simulink model "sim_inverted_pendulum_atrito2"  (R2018a)
settings: Solver=FixedStepAuto  StartTime=0.0  StopTime=30  FixedStep=1e-3  RelTol=1e-3
model workspace (MAT data in the model file):
  Ts = 0.01
values from neighbouring files (symbols this model uses):
  bl = 1*3    (= 3)    [param.m]
  br = 1*1.25    (= 1.25)    [param.m]
  g = 9.8    [param.m]
  L = 1.5    [param.m]
  M = 2    [param.m]
  m = 0.5    [param.m]
libraries: simulink x2
settings Model: Creator=ederm  LastModifiedBy=isabe

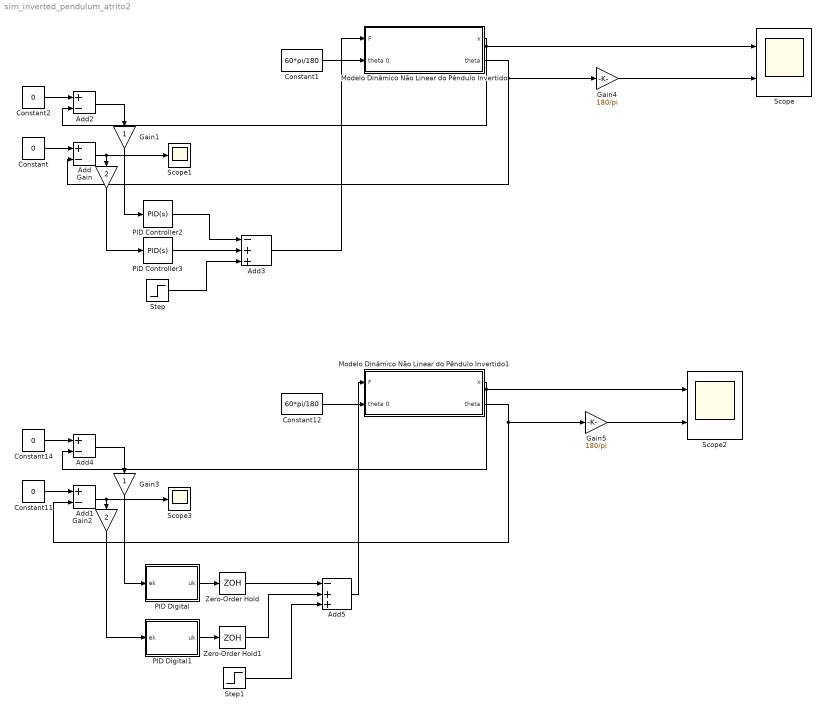
== system sim_inverted_pendulum_atrito2 ==
  Add{,1..2,4} (4 alike) : Sum  Inputs=+-
  Add3 : Sum  Inputs=-++
  Add5 : Sum  Inputs=-++
  Constant{,2,11,14} (4 alike) : Constant  Value=0
  Constant1 : Constant  Value=60*pi/180
  Constant12 : Constant  Value=60*pi/180
  Gain : Gain  Gain=2
  Gain1 : Gain
  Gain2 : Gain  Gain=2
  Gain3 : Gain
  Gain4 : Gain  Gain=180/pi
  Gain5 : Gain  Gain=180/pi
  Modelo Dinâmico Não Linear do Pêndulo Invertido : Subsystem
  Modelo Dinâmico Não Linear do Pêndulo Invertido1 : Subsystem
  PID Controller2 : simulink/Continuous/PID Controller  Controller=PID  TimeDomain=Continuous-time  SampleTime=-1  IntegratorMethod=Forward Euler  FilterMethod=Forward Euler  Form=Parallel  UseFilter=on  ControllerParametersSource=internal  P=10  I=2.5  D=1.4  N=100  InitialConditionSource=internal  InitialConditionForIntegrator=0  InitialConditionForFilter=0  ExternalReset=none  LimitOutput=off  UpperSaturationLimit=inf  LowerSaturationLimit=-inf  LinearizeAsGain=on  AntiWindupMode=none  Kb=1  TrackingMode=off  Kt=1  PParamMin=[]  PParamMax=[]  IParamMin=[]  IParamMax=[]  DParamMin=[]  DParamMax=[]  NParamMin=[]  NParamMax=[]  KbParamMin=[]  KbParamMax=[]  KtParamMin=[]  KtParamMax=[]  POutMin=[]  POutMax=[]  IOutMin=[]  IOutMax=[]  DOutMin=[]  DOutMax=[]  NOutMin=[]  NOutMax=[]  KbOutMin=[]  KbOutMax=[]  KtOutMin=[]  KtOutMax=[]  IntegratorOutMin=[]  IntegratorOutMax=[]  FilterOutMin=[]  FilterOutMax=[]  SumOutMin=[]  SumOutMax=[]  SumI1OutMin=[]  SumI1OutMax=[]  SumI2OutMin=[]  SumI2OutMax=[]  SumI3OutMin=[]  SumI3OutMax=[]  SumDOutMin=[]  SumDOutMax=[]  SaturationOutMin=[]  SaturationOutMax=[]  IntegratorContinuousStateAttributes=''  IntegratorStateMustResolveToSignalObject=off  IntegratorRTWStateStorageClass=Auto  FilterContinuousStateAttributes=''  FilterStateMustResolveToSignalObject=off  FilterRTWStateStorageClass=Auto  DifferentiatorICPrevScaledInput=0  DifferentiatorOutMin=[]  DifferentiatorOutMax=[]  FilterDiffOutCoefMin=[]  FilterDiffOutCoefMax=[]  SumDenOutMin=[]  SumDenOutMax=[]  SumNumOutMin=[]  SumNumOutMax=[]  ReciprocalOutMin=[]  ReciprocalOutMax=[]  DivideOutMin=[]  DivideOutMax=[]  TunerSelectOption=Transfer Function Based (PID Tuner App)
  PID Controller3 : simulink/Continuous/PID Controller  Controller=PID  TimeDomain=Continuous-time  SampleTime=-1  IntegratorMethod=Forward Euler  FilterMethod=Forward Euler  Form=Parallel  UseFilter=on  ControllerParametersSource=internal  P=70  I=110  D=12  N=100  InitialConditionSource=internal  InitialConditionForIntegrator=0  InitialConditionForFilter=0  ExternalReset=none  LimitOutput=off  UpperSaturationLimit=inf  LowerSaturationLimit=-inf  LinearizeAsGain=on  AntiWindupMode=none  Kb=1  TrackingMode=off  Kt=1  PParamMin=[]  PParamMax=[]  IParamMin=[]  IParamMax=[]  DParamMin=[]  DParamMax=[]  NParamMin=[]  NParamMax=[]  KbParamMin=[]  KbParamMax=[]  KtParamMin=[]  KtParamMax=[]  POutMin=[]  POutMax=[]  IOutMin=[]  IOutMax=[]  DOutMin=[]  DOutMax=[]  NOutMin=[]  NOutMax=[]  KbOutMin=[]  KbOutMax=[]  KtOutMin=[]  KtOutMax=[]  IntegratorOutMin=[]  IntegratorOutMax=[]  FilterOutMin=[]  FilterOutMax=[]  SumOutMin=[]  SumOutMax=[]  SumI1OutMin=[]  SumI1OutMax=[]  SumI2OutMin=[]  SumI2OutMax=[]  SumI3OutMin=[]  SumI3OutMax=[]  SumDOutMin=[]  SumDOutMax=[]  SaturationOutMin=[]  SaturationOutMax=[]  IntegratorContinuousStateAttributes=''  IntegratorStateMustResolveToSignalObject=off  IntegratorRTWStateStorageClass=Auto  FilterContinuousStateAttributes=''  FilterStateMustResolveToSignalObject=off  FilterRTWStateStorageClass=Auto  DifferentiatorICPrevScaledInput=0  DifferentiatorOutMin=[]  DifferentiatorOutMax=[]  FilterDiffOutCoefMin=[]  FilterDiffOutCoefMax=[]  SumDenOutMin=[]  SumDenOutMax=[]  SumNumOutMin=[]  SumNumOutMax=[]  ReciprocalOutMin=[]  ReciprocalOutMax=[]  DivideOutMin=[]  DivideOutMax=[]  TunerSelectOption=Transfer Function Based (PID Tuner App)
  PID Digital : MATLAB Function  TreatAsAtomicUnit=on  SystemSampleTime=Ts
  PID Digital1 : MATLAB Function  TreatAsAtomicUnit=on  SystemSampleTime=Ts
  Scope : Scope  NumInputPorts=2
  Scope1 : Scope
  Scope2 : Scope  NumInputPorts=2
  Scope3 : Scope
  Step : Step  Time=10  After=3  SampleTime=0
  Step1 : Step  Time=10  After=3  SampleTime=0
  Zero-Order Hold : ZeroOrderHold  SampleTime=-1
  Zero-Order Hold1 : ZeroOrderHold  SampleTime=-1
  wires:
  Modelo Dinâmico Não Linear do Pêndulo Invertido/1(x) -> Add2/2, Scope/1
  Constant/1 -> Add/1
  Constant1/1 -> Modelo Dinâmico Não Linear do Pêndulo Invertido/2(theta 0)
  Constant2/1 -> Add2/1
  Add2/1 -> Gain1/1
  Step/1 -> Add3/3
  Add3/1 -> Modelo Dinâmico Não Linear do Pêndulo Invertido/1(F)
  Modelo Dinâmico Não Linear do Pêndulo Invertido/2(theta) -> Add/2, Gain4/1
  Add/1 -> Scope1/1, Gain/1
  Gain/1 -> PID Controller3/1
  Gain1/1 -> PID Controller2/1
  Gain3/1 -> PID Digital/1(ek)
  Step1/1 -> Add5/3
  Gain2/1 -> PID Digital1/1(ek)
  Modelo Dinâmico Não Linear do Pêndulo Invertido1/1(x) -> Add4/2, Scope2/1
  Constant12/1 -> Modelo Dinâmico Não Linear do Pêndulo Invertido1/2(theta 0)
  Constant11/1 -> Add1/1
  Add5/1 -> Modelo Dinâmico Não Linear do Pêndulo Invertido1/1(F)
  Add1/1 -> Scope3/1, Gain2/1
  Constant14/1 -> Add4/1
  Add4/1 -> Gain3/1
  Zero-Order Hold/1 -> Add5/1
  Zero-Order Hold1/1 -> Add5/2
  Modelo Dinâmico Não Linear do Pêndulo Invertido1/2(theta) -> Add1/2, Gain5/1
  PID Digital1/1(uk) -> Zero-Order Hold1/1
  PID Controller2/1 -> Add3/1
  PID Controller3/1 -> Add3/2
  Gain4/1 -> Scope/2
  Gain5/1 -> Scope2/2
  PID Digital/1(uk) -> Zero-Order Hold/1

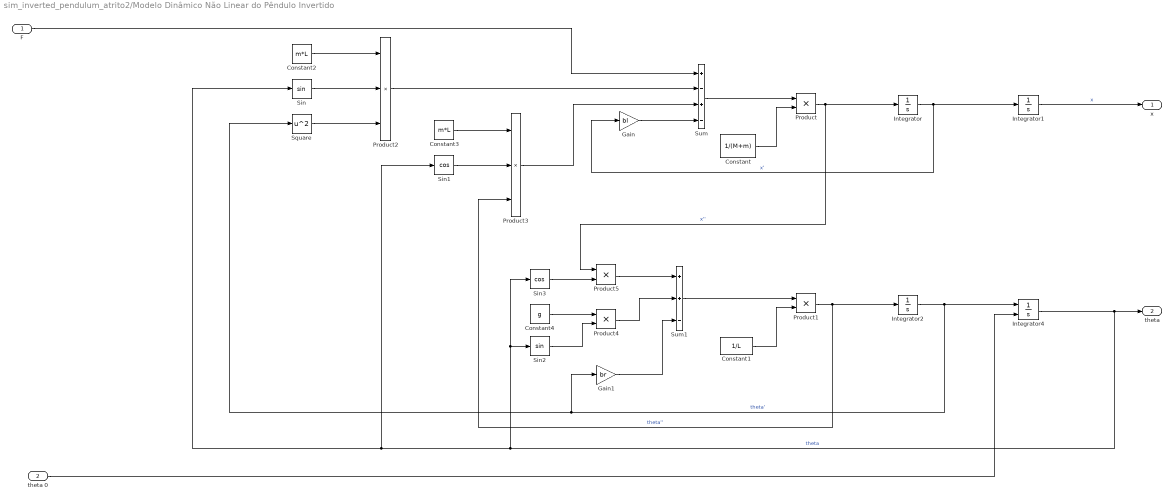
== system sim_inverted_pendulum_atrito2/Modelo Dinâmico Não Linear do Pêndulo Invertido ==
  F : Inport
  theta 0 : Inport  Port=2
  Constant : Constant  Value=1/(M+m)
  Constant1 : Constant  Value=1/L
  Constant2 : Constant  Value=m*L
  Constant3 : Constant  Value=m*L
  Constant4 : Constant  Value=g
  Gain : Gain  Gain=bl
  Gain1 : Gain  Gain=br
  Integrator : Integrator
  Integrator1 : Integrator
  Integrator2 : Integrator
  Integrator4 : Integrator  InitialConditionSource=external
  Product{,1,4..5} (4 alike) : Product
  Product2 : Product  Inputs=3
  Product3 : Product  Inputs=3
  Sin : Trigonometry
  Sin1 : Trigonometry  Operator=cos
  Sin2 : Trigonometry
  Sin3 : Trigonometry  Operator=cos
  Square : Math  Operator=square  SaturateOnIntegerOverflow=on
  Sum : Sum  Inputs=+-+-
  Sum1 : Sum  Inputs=++-
  x : Outport
  theta : Outport  Port=2
  wires:
  Product1/1 -> Product3/3, Integrator2/1  "theta''"
  Integrator/1 -> Gain/1, Integrator1/1  "x'"
  Sum/1 -> Product/1
  Constant2/1 -> Product2/1
  Constant3/1 -> Product3/1
  Integrator2/1 -> Gain1/1, Square/1, Integrator4/1  "theta'"
  Integrator4/1 -> theta/1, Sin3/1, Sin2/1, Sin1/1, Sin/1  "theta"
  Product4/1 -> Sum1/2
  Gain1/1 -> Sum1/3
  Constant1/1 -> Product1/2
  Constant4/1 -> Product4/1
  Sin2/1 -> Product4/2
  Product3/1 -> Sum/3
  Product/1 -> Product5/1, Integrator/1  "x''"
  Sin3/1 -> Product5/2
  Sum1/1 -> Product1/1
  F/1 -> Sum/1
  Product5/1 -> Sum1/1
  Product2/1 -> Sum/2
  Gain/1 -> Sum/4
  Sin/1 -> Product2/2
  Constant/1 -> Product/2
  Square/1 -> Product2/3
  Sin1/1 -> Product3/2
  Integrator1/1 -> x/1  "x"
  theta 0/1 -> Integrator4/2

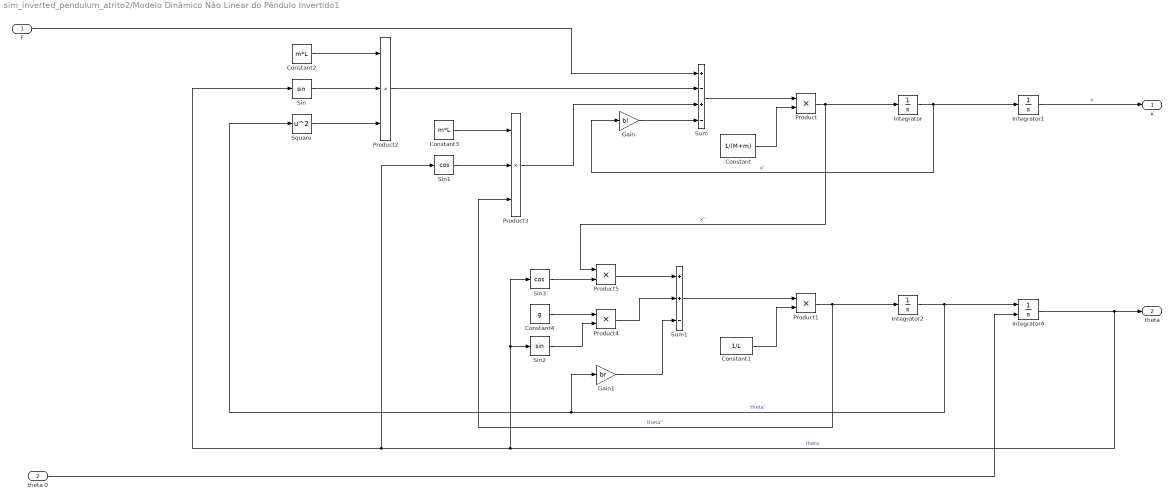
== system sim_inverted_pendulum_atrito2/Modelo Dinâmico Não Linear do Pêndulo Invertido1 ==
  F : Inport
  theta 0 : Inport  Port=2
  Constant : Constant  Value=1/(M+m)
  Constant1 : Constant  Value=1/L
  Constant2 : Constant  Value=m*L
  Constant3 : Constant  Value=m*L
  Constant4 : Constant  Value=g
  Gain : Gain  Gain=bl
  Gain1 : Gain  Gain=br
  Integrator : Integrator
  Integrator1 : Integrator
  Integrator2 : Integrator
  Integrator4 : Integrator  InitialConditionSource=external
  Product{,1,4..5} (4 alike) : Product
  Product2 : Product  Inputs=3
  Product3 : Product  Inputs=3
  Sin : Trigonometry
  Sin1 : Trigonometry  Operator=cos
  Sin2 : Trigonometry
  Sin3 : Trigonometry  Operator=cos
  Square : Math  Operator=square  SaturateOnIntegerOverflow=on
  Sum : Sum  Inputs=+-+-
  Sum1 : Sum  Inputs=++-
  x : Outport
  theta : Outport  Port=2
  wires:
  Product1/1 -> Product3/3, Integrator2/1  "theta''"
  Integrator/1 -> Gain/1, Integrator1/1  "x'"
  Sum/1 -> Product/1
  Constant2/1 -> Product2/1
  Constant3/1 -> Product3/1
  Integrator2/1 -> Gain1/1, Square/1, Integrator4/1  "theta'"
  Integrator4/1 -> theta/1, Sin3/1, Sin2/1, Sin1/1, Sin/1  "theta"
  Product4/1 -> Sum1/2
  Gain1/1 -> Sum1/3
  Constant1/1 -> Product1/2
  Constant4/1 -> Product4/1
  Sin2/1 -> Product4/2
  Product3/1 -> Sum/3
  Product/1 -> Product5/1, Integrator/1  "x''"
  Sin3/1 -> Product5/2
  Sum1/1 -> Product1/1
  F/1 -> Sum/1
  Product5/1 -> Sum1/1
  Product2/1 -> Sum/2
  Gain/1 -> Sum/4
  Sin/1 -> Product2/2
  Constant/1 -> Product/2
  Square/1 -> Product2/3
  Sin1/1 -> Product3/2
  Integrator1/1 -> x/1  "x"
  theta 0/1 -> Integrator4/2

== matlab function sim_inverted_pendulum_atrito2/PID Digital1 ==
  data: ek input; uk output
function uk = fcn(ek)

persistent ek_1 ek_sum

if isempty(ek_1)
    ek_1 = 0;
    ek_sum = 0;
end

Ts = 0.01;

Kp = 70;
Ki = 110;
Kd = 12; 

ek_sum = Ts*ek + ek_sum;

uk = Kp * ek + ...
     Ki * (ek_sum) + ...
     (Kd/Ts) * (ek - ek_1);

ek_1 = ek

== matlab function sim_inverted_pendulum_atrito2/PID Digital ==
  data: ek input; uk output
function uk = fcn(ek)

Ts = 0.01;

persistent ek_1 ek_sum

if isempty(ek_1)
    ek_1 = 0;
    ek_sum = 0;
end

Kp = 10; 
Ki = 2.4;
Kd = 1.4; 

ek_sum = Ts*ek + ek_sum;

uk = Kp * ek + ...
     Ki * (ek_sum) + ...
     (Kd/Ts) * (ek - ek_1);

ek_1 = ek
